simulink model "GNCsimulator_MoonOrbit"  (R2023b)
settings: Solver=ode113  StartTime=0.0  StopTime=1000  FixedStep=1  RelTol=1e-13  AbsTol=1e-13
values from neighbouring files (symbols this model uses):
  bENABLE_3rdBodyAccel_EARTH = true    [simMain_MoonOrbit.m]
  bENABLE_3rdBodyAccel_SUN = true    [simMain_MoonOrbit.m]
  bENABLE_3rdBodyAccel_VENUS = false    [simMain_MoonOrbit.m]
  bENABLE_CannonBallSRPaccel = true    [simMain_MoonOrbit.m]
  bENABLE_SHE_MOON = true    [simMain_MoonOrbit.m]
  xSCref0 = kepl2rv(SatID5A_keplParams, mu_Moon)    [simMain_MoonOrbit.m]
libraries: orbitalModelsLib x8, sensorsModelsLib x1
settings Model: Creator=pietr  LastModifiedBy=pietr
settings SolverCC: ShapePreserveControl=EnableAll  ZeroCrossAlgorithm=Adaptive  AutoInsertRateTranBlk=on  InsertRTBMode=Always  DecoupledContinuousIntegration=on  MinimalZcImpactIntegration=on
settings OptimizationCC: ReuseModelBlockBuffer=off

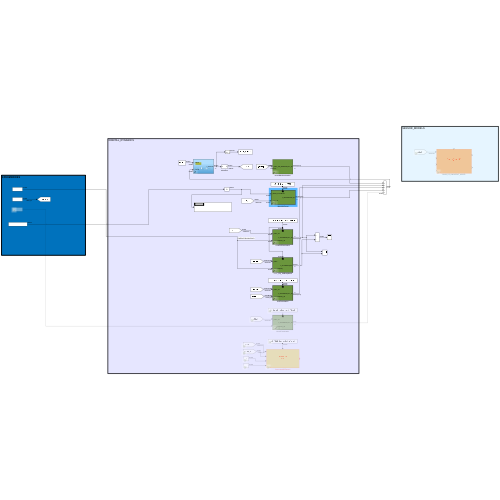
[thumbnail: Simulink's stored preview of the top-level diagram]
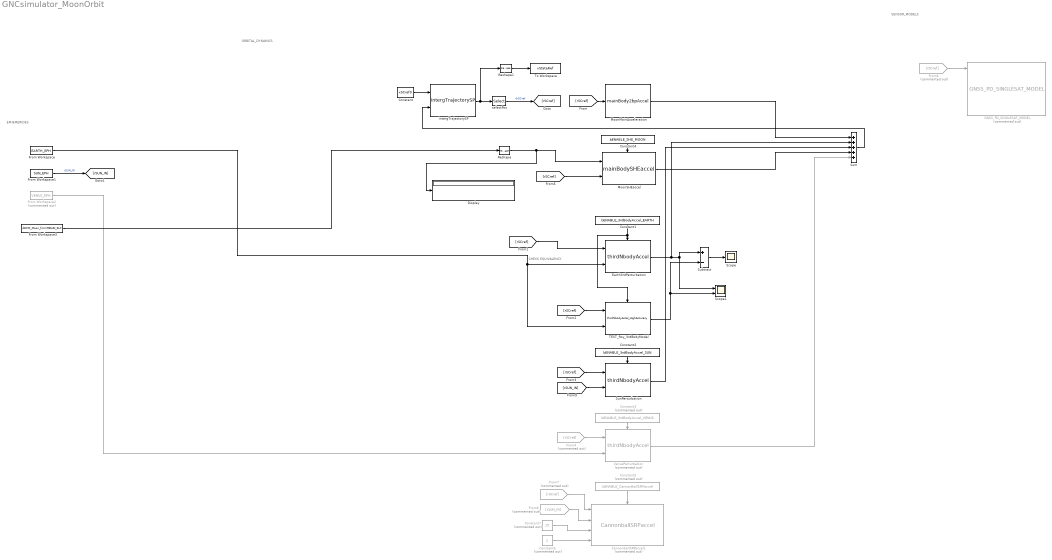
== system GNCsimulator_MoonOrbit ==
  note: EPHEMERIDES
  note: SENSOR_MODELS
  note: CHECK EQUIVALENCY
  note: ORBITAL_DYNAMICS
  CannonballSRPaccel1 : orbitalModelsLib/CannonballSRPaccel  Commented=on  ReflCoeffParam=dReflectivityCoeff
      settings: SourceProductName=orbitalModelsLib
  Constant : Constant  Value=xSCref0
  Constant1 : Constant  Value=bENABLE_3rdBodyAccel_EARTH  OutDataTypeStr=boolean
  Constant2 : Constant  Value=bENABLE_3rdBodyAccel_SUN  OutDataTypeStr=boolean
  Constant3 : Constant  Commented=on  Value=bENABLE_3rdBodyAccel_VENUS  OutDataTypeStr=boolean
  Constant4 : Constant  Value=bENABLE_SHE_MOON  OutDataTypeStr=boolean
  Constant5 : Constant  Commented=on  Value=bENABLE_CannonBallSRPaccel  OutDataTypeStr=boolean
  Constant6 : Constant  Commented=on
  Constant7 : Constant  Commented=on  Value=15
  Display : Display
  Earth3rdPerturbation : orbitalModelsLib/thirdNbodyAccel  MuBody=mu_Earth
      settings: SourceProductName=orbitalModelsLib
  From Workspace : FromWorkspace  VariableName=EARTH_EPH  OutputAfterFinalValue=Holding final value
  From Workspace1 : FromWorkspace  VariableName=SUN_EPH  OutputAfterFinalValue=Holding final value
  From Workspace2 : FromWorkspace  Commented=on  VariableName=VENUS_EPH  OutputAfterFinalValue=Holding final value
  From Workspace3 : FromWorkspace  VariableName=dDCM_Moon_fromTBtoIN_SLX  Interpolate=off  OutputAfterFinalValue=Holding final value
  From4 : From  Commented=on  GotoTag=rSCref
  From6 : From  Commented=on  GotoTag=rSCref
  From7 : From  Commented=on  GotoTag=rSCref
  From8 : From  Commented=on  GotoTag=rSUN_IN
  GNSS_PD_SINGLESAT_MODEL : sensorsModelsLib/GNSS_PD_SINGLESAT_MODEL  Commented=on  bGNSS_2CLOCKNOISE_MODEL=bGNSS_2CLOCKNOISE_MODEL  EnableRangeWN=bENABLE_WN  EnableRangeRateWN=bENABLE_WN  BiasMean=0  BiasSeed=0  BiasVar=1  DriftMean=0  DriftSeed=0  DriftVar=1  VarRangeRateWN=1  RNGseedRangeRateWN=0  MeanRangeRateWN=0  VarRangeWN=1  RNGseedRangeWN=0  MeanRangeWN=0
  MoonMainAcceleration : orbitalModelsLib/mainBody2bpAccel  MuBody=mu_Moon_SHref
      settings: SourceProductName=orbitalModelsLib
  MoonSHEaccel : orbitalModelsLib/mainBodySHEaccel  GravParam=mu_Moon_SHref  ClmSlm_unnormalized=i_dCSlmCoeffCols  BodyRref=R_Moon_SHref  MaxSHdegree=maxSHEdegree
      settings: SourceProductName=orbitalModelsLib
  Reshape : Reshape  OutputDimensionality=Customize  OutputDimensions=[3, 3]
  Reshape1 : Reshape
  Scope : Scope
  Scope1 : Scope  NumInputPorts=2
  Subtract : Sum  Inputs=+-
  Sum : Sum  Inputs=+++++
  SunPerturbation : orbitalModelsLib/thirdNbodyAccel  MuBody=mu_Sun
      settings: SourceProductName=orbitalModelsLib
  TEST_Roy_3rdBodyModel : orbitalModelsLib/thirdNbodyAccel_HighAccuracy  MuBody=mu_Earth
      settings: SourceProductName=orbitalModelsLib
  To Workspace : ToWorkspace  VariableName=xStateRef  SaveFormat=Timeseries  SampleTime=1
  VenusPerturbation : orbitalModelsLib/thirdNbodyAccel  Commented=on  MuBody=mu
      settings: SourceProductName=orbitalModelsLib
  intergTrajectorySP : orbitalModelsLib/intergTrajectorySP  SystemSampleTime=-1  VariantActivationTime=update diagram  AllowFlexibleInterface=on  Latency=0  AutoFrameSizeCalculation=off
      settings: SourceProductName=orbitalModelsLib
  selectPos : Selector  InputPortWidth=6  IndexOptions=Index vector (dialog)  Indices=[1:3]  OutputSizes=1
  wires:
  MoonMainAcceleration/1 -> Sum/1
  Earth3rdPerturbation/1 -> Scope1/1, Subtract/1, Sum/2
  intergTrajectorySP/1 -> selectPos/1, Reshape1/1
  TEST_Roy_3rdBodyModel/1 -> Subtract/2, Scope1/2
  Subtract/1 -> Scope/1
  Sum/1 -> intergTrajectorySP/2
  Constant/1 -> intergTrajectorySP/1
  Constant1/1 -> TEST_Roy_3rdBodyModel/Enable, Earth3rdPerturbation/Enable
  From Workspace/1 -> TEST_Roy_3rdBodyModel/2, Earth3rdPerturbation/2
  selectPos/1 -> [rSCref]  "drSCref"
  [rSCref] -> MoonMainAcceleration/1
  [rSCref] -> Earth3rdPerturbation/1
  [rSCref] -> TEST_Roy_3rdBodyModel/1
  [rSCref] -> SunPerturbation/1
  Constant2/1 -> SunPerturbation/Enable
  SunPerturbation/1 -> Sum/3
  From4/1 -> VenusPerturbation/1
  From Workspace2/1 -> VenusPerturbation/2
  Constant4/1 -> MoonSHEaccel/Enable
  MoonSHEaccel/1 -> Sum/4
  VenusPerturbation/1 -> Sum/5
  [rSCref] -> MoonSHEaccel/2
  Constant3/1 -> VenusPerturbation/Enable
  From Workspace3/1 -> Reshape/1
  Reshape/1 -> Display/1, MoonSHEaccel/1
  Reshape1/1 -> To Workspace/1
  From6/1 -> GNSS_PD_SINGLESAT_MODEL/1
  Constant6/1 -> CannonballSRPaccel1/4
  Constant5/1 -> CannonballSRPaccel1/Enable
  Constant7/1 -> CannonballSRPaccel1/3
  From8/1 -> CannonballSRPaccel1/2
  From7/1 -> CannonballSRPaccel1/1
  [rSUN_IN] -> SunPerturbation/2
  From Workspace1/1 -> [rSUN_IN]  "rSUN_IN"
